simulink model "dr_can_calorie_pi"  (R2022a)
settings: Solver=VariableStepAuto  StartTime=0.0  StopTime=500  RelTol=1e-3
libraries: cstblocks x1
settings Model: Creator=pw705  LastModifiedBy=pw705

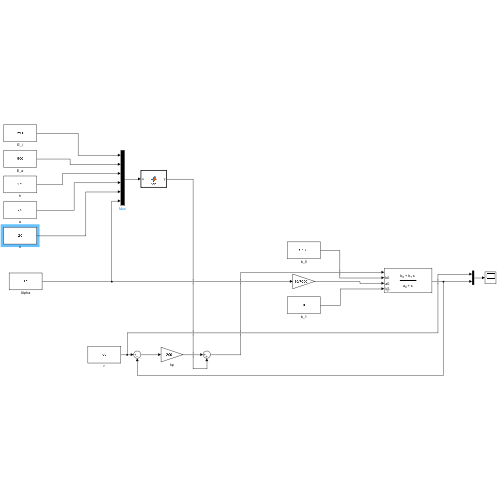
[thumbnail: Simulink's stored preview of the top-level diagram]
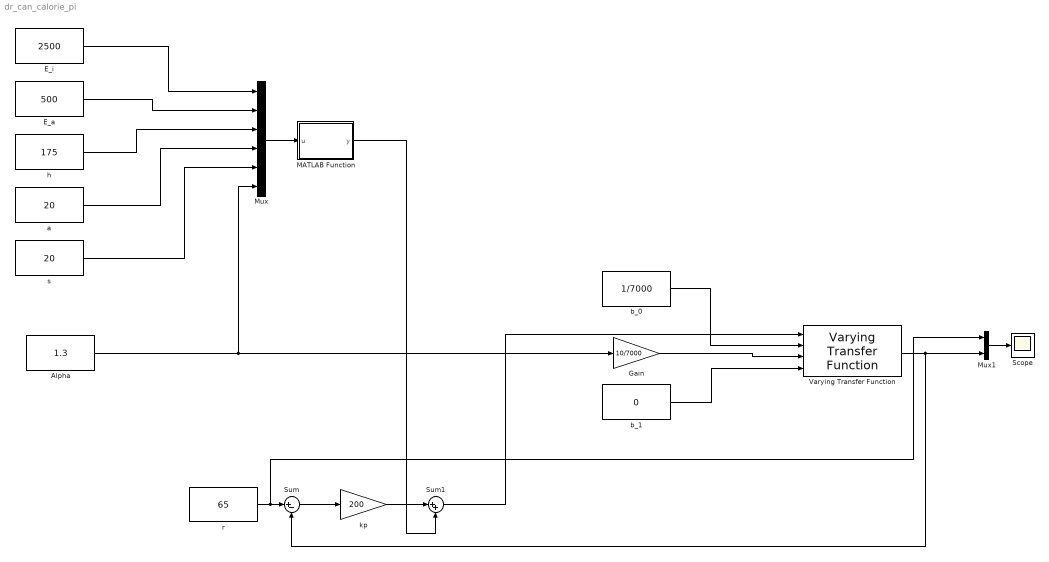
== system dr_can_calorie_pi ==
  Alpha : Constant  Value=1.3
  E_a : Constant  Value=500
  E_i : Constant  Value=2500
  Gain : Gain  Gain=10/7000
  MATLAB Function : MATLAB Function  TreatAsAtomicUnit=on
  Mux : Mux  Inputs=6
  Mux1 : Mux  Inputs=2
  Scope : Scope
  Sum : Sum  Inputs=|+-
  Sum1 : Sum  Inputs=|++
  Varying Transfer Function : cstblocks/Linear Parameter Varying/Varying Transfer Function  N=1
      link override Integrator1: InitialCondition=70
  a : Constant  Value=20
  b_0 : Constant  Value=1/7000
  b_1 : Constant  Value=0
  h : Constant  Value=175
  kp : Gain  Gain=200
  r : Constant  Value=65
  s : Constant  Value=20
  wires:
  b_0/1 -> Varying Transfer Function/2
  Alpha/1 -> Gain/1, Mux/6
  Gain/1 -> Varying Transfer Function/3
  b_1/1 -> Varying Transfer Function/4
  MATLAB Function/1(y) -> Sum1/2
  E_i/1 -> Mux/1
  E_a/1 -> Mux/2
  h/1 -> Mux/3
  a/1 -> Mux/4
  s/1 -> Mux/5
  Mux/1 -> MATLAB Function/1(u)
  Varying Transfer Function/1 -> Mux1/2, Sum/2
  Sum/1 -> kp/1
  kp/1 -> Sum1/1
  Sum1/1 -> Varying Transfer Function/1
  r/1 -> Mux1/1, Sum/1
  Mux1/1 -> Scope/1

== matlab function dr_can_calorie_pi/MATLAB Function ==
  data: u input; y output
function y = fcn(u)
    

y = u(1)-u(2)-u(6)*(6.25*u(3)-5*u(4)+u(5));
